simulink model "test"  (R2023a)
settings: Solver=ode1  StartTime=0.0  StopTime=inf  FixedStep=0.002  RelTol=1e-3  EnableMultiTasking=on
undefined symbols (not defined in the file or in its folder): HIL
libraries: quarc_library x18, simulink x1
settings Model: ExtModeTrigDuration=10000  Creator=bajdus  LastModifiedBy=bajdus
settings SolverCC: AlgebraicLoopSolver=TrustRegion  PositivePriorityOrder=on
settings DataIOCC: ReturnWorkspaceOutputs=off
settings DebuggingCC: UnconnectedInputMsg=warning  UnconnectedOutputMsg=warning  UnconnectedLineMsg=warning  ArithmeticOperatorsInVariantConditions=warning
settings HardwareCC: ProdBitPerLong=64  ProdLargestAtomicInteger=LongLong  ProdLargestAtomicFloat=Double  ProdLongLongMode=on  ProdHWDeviceType=ARM Compatible->ARM 64-bit (LP64)
settings ModelReferenceCC: EnableRefExpFcnMdlSchedulingChecks=on
settings SFSimCC: SimUseLocalCustomCode=off  CustomCodeUndefinedFunction=UseInterfaceOnly
settings RTWCC: Description=QUARC Linux QCar2 Target Using Toolchain  SystemTargetFile=quarc_linux_qcar2.tlc  TemplateMakefile=quarc_default_tmf  RTWUseLocalCustomCode=off  Toolchain=QUARC linux_qcar2 | gmake (64-bit Windows)  BuildConfiguration=Faster Runs
settings CodeAppCC: StateflowObjectComments=on
settings STFCustomTargetCC: SystemTargetFile=quarc_linux_qcar2.tlc
settings GRTTargetCC: ParMdlRefBuildCompliant=off  CompOptLevelCompliant=off  CombineOutputUpdateFcns=off  MatFileLogging=off  CPPClassGenCompliant=off  GRTInterface=on  ExtMode=on  ExtModeMexFile=quarc_comm  ExtModeMexArgs='-w -d /tmp -uri %u', 'tcpip://192.168.1.126:17001'
settings ConfigComp: CovMetricSettings=dswe

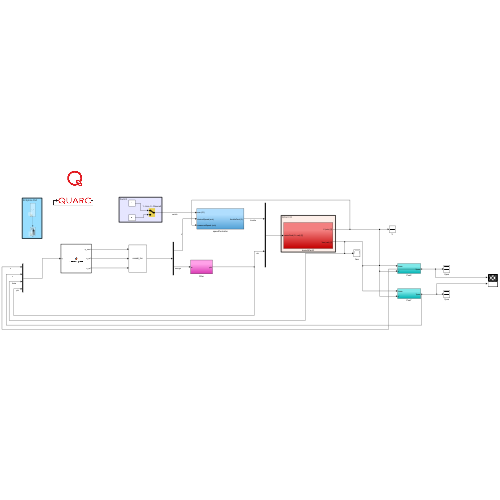
[thumbnail: Simulink's stored preview of the top-level diagram]
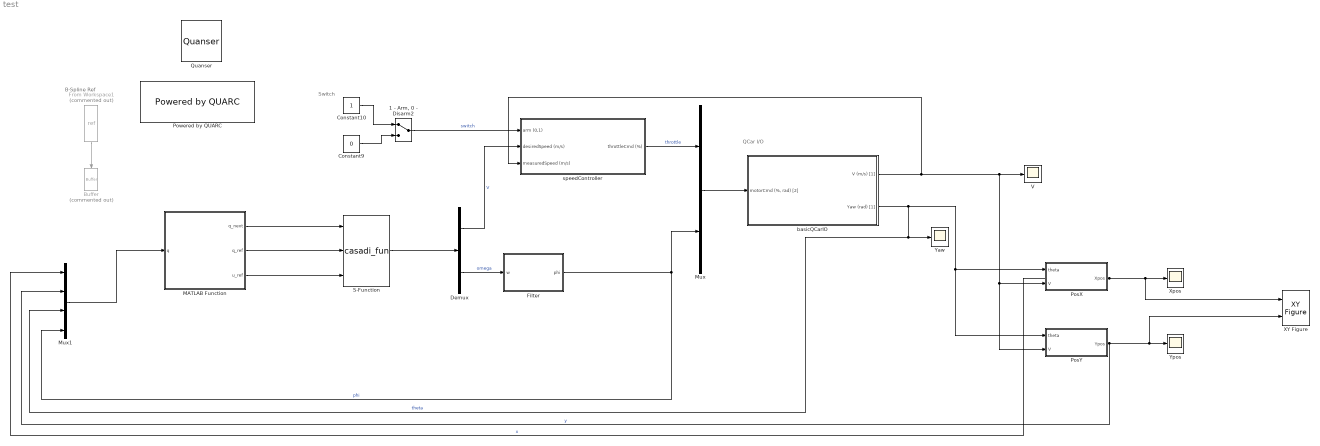
== system test ==
  note: QCar I/O
  note: Switch
  note: B-Spline Ref
  "1 - Arm, 0 - Disarm2" : ManualSwitch
  Buffer : Buffer  Commented=on  N=54  OutputFrames=off
  Constant10 : Constant
  Constant9 : Constant  Value=0
  Demux : Demux  Outputs=2
  Filter : Subsystem
  From Workspace1 : FromWorkspace  Commented=on  VariableName=ref  SampleTime=0.1  ZeroCross=off
  MATLAB Function : MATLAB Function  TreatAsAtomicUnit=on
  Mux : Mux  Inputs=2
  Mux1 : Mux
  PosX : Subsystem
  PosY : Subsystem
  Powered by QUARC : quarc_library/Logos/Powered by QUARC
  Quanser : quarc_library/Logos/Quanser
  S-Function : S-Function  FunctionName=casadi_fun  Parameters='nmpc_oncar.casadi','nmpc_oncar'  SFunctionDeploymentMode=off  EnableBusSupport=off
  V : Scope
  XY Figure : quarc_library/Sinks/Figures/XY Figure  figure_mode=Use figure window  figure_tag=figure1  axes_tag=axes1  plot_mode=Time-based  minimum_x=-5  maximum_x=5  minimum_y=-5  maximum_y=5  buffer_size=1000000  update_rate=100  initial_position="1.8          41.8         439.2         331.2"  initial_visibility=off  sample_time=-1
      settings: SourceProductName=QUARC Targets
  Xpos : Scope
  Yaw : Scope
  Ypos : Scope
  basicQCarIO : Subsystem
  speedController : Subsystem
  wires:
  Mux/1 -> basicQCarIO/1("motorCmd (%, rad) [2]")
  "1 - Arm, 0 - Disarm2"/1 -> speedController/1(arm (0,1))  "switch"
  Constant10/1 -> "1 - Arm, 0 - Disarm2"/1
  speedController/1(throttleCmd (%)) -> Mux/1  "throttle"
  basicQCarIO/1(V (m/s) [1]) -> speedController/3(measuredSpeed (m/s)), V/1, PosX/2(V), PosY/2(V)
  Constant9/1 -> "1 - Arm, 0 - Disarm2"/2
  PosX/1(Xpos) -> XY Figure/1, Xpos/1, Mux1/1  "x"
  PosY/1(Ypos) -> XY Figure/2, Ypos/1, Mux1/2  "y"
  basicQCarIO/2(Yaw (rad) [1]) -> Mux1/3, Yaw/1, PosY/1(theta), PosX/1(theta)  "theta"
  Filter/1(phi) -> Mux1/4, Mux/2  "phi"
  Demux/1 -> speedController/2(desiredSpeed (m/s))  "V"
  Demux/2 -> Filter/1(w)  "omega"
  From Workspace1/1 -> Buffer/1
  Mux1/1 -> MATLAB Function/1(q)
  S-Function/1 -> Demux/1
  MATLAB Function/1(q_next) -> S-Function/1
  MATLAB Function/2(q_ref) -> S-Function/2
  MATLAB Function/3(u_ref) -> S-Function/3

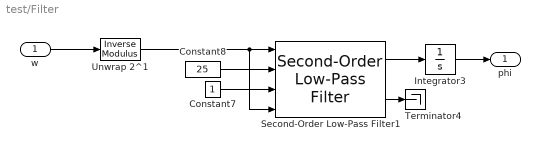
== system test/Filter ==
  w : Inport
  Constant7 : Constant
  Constant8 : Constant  Value=25
  Integrator3 : Integrator
  Second-Order Low-Pass Filter1 : quarc_library/Continuous/Second-Order Low-Pass Filter  params_source=External (input ports)  input_width=1  input_zeta=1  input_init=0
  Terminator4 : Terminator
  Unwrap 2^1 : quarc_library/Discontinuities/Inverse Modulus  modulus=16777215  output_derivative=off  output_revolutions=off  max_x=Inf  min_x=-Inf
  phi : Outport
  wires:
  Constant8/1 -> Second-Order Low-Pass Filter1/2
  Constant7/1 -> Second-Order Low-Pass Filter1/3
  Second-Order Low-Pass Filter1/1 -> Integrator3/1
  Unwrap 2^1/1 -> Second-Order Low-Pass Filter1/4, Second-Order Low-Pass Filter1/1
  w/1 -> Unwrap 2^1/1
  Second-Order Low-Pass Filter1/2 -> Terminator4/1
  Integrator3/1 -> phi/1

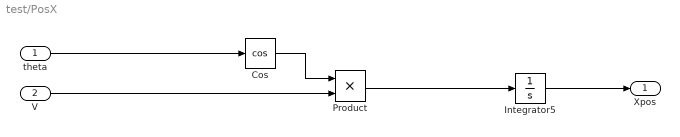
== system test/PosX ==
  theta : Inport
  V : Inport  Port=2
  Cos : Trigonometry  Operator=cos
  Integrator5 : Integrator
  Product : Product
  Xpos : Outport
  wires:
  Cos/1 -> Product/1
  theta/1 -> Cos/1
  V/1 -> Product/2
  Integrator5/1 -> Xpos/1
  Product/1 -> Integrator5/1

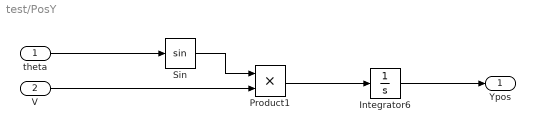
== system test/PosY ==
  theta : Inport
  V : Inport  Port=2
  Integrator6 : Integrator
  Product1 : Product
  Sin : Trigonometry
  Ypos : Outport
  wires:
  theta/1 -> Sin/1
  V/1 -> Product1/2
  Sin/1 -> Product1/1
  Integrator6/1 -> Ypos/1
  Product1/1 -> Integrator6/1

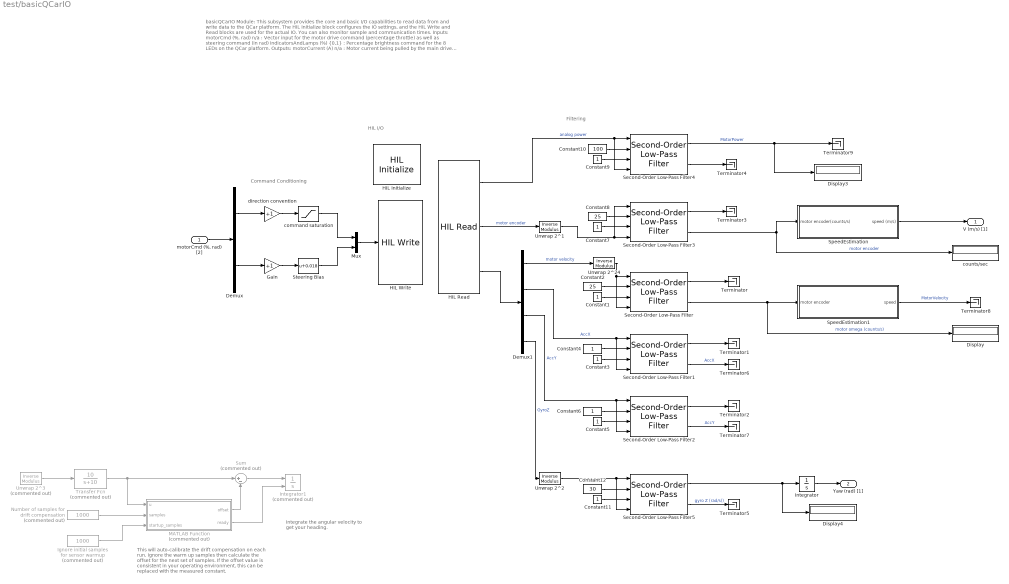
== system test/basicQCarIO ==
  note: Filtering
  note: basicQCarIO Module:
      |
      | This subsystem provides the core and basic I/O capabilities to read data from and write data to the QCar platform. The HIL Initialize block configures the IO settings, and the HIL Write and Read blocks are used for the actual IO. You can also monitor sample and communication times.
      |
      | Inputs:
      | motorCmd (%, rad) n/a : Vector input for the motor drive command (percentage throttle) as well as steering command (in rad)
      | indicatorsAndLamps (%) {0,1} : Percentage brightness command for the 8 LEDs on the QCar platform.
      |
      | Outputs:
      | motorCurrent (A) n/a : Motor current being pulled by the main drive motor
      | batteryVoltage (V) {0, 12.6} : Current battery voltage reading
      | motorSpeed (counts/s) n/a : Drive motor speed measured using an encoder (do not confuse with wheel speed as this measurement is at the drive shaft)
  note: Command Conditioning
  note: HIL I/O
  note: Integrate the angular velocity to
      | get your heading.
  note: This will auto-calibrate the drift compensation
      | on each run. Ignore the warm up samples
      | then calculate the offset for the next set of samples.
      | If the offset value is consistent in your operating
      | environment, this can be replaced with the measured
      | constant.
  "motorCmd (%, rad) [2]" : Inport
  Constant{1,3..7,9,11} (8 alike) : Constant
  Constant10 : Constant  Value=100
  Constant12 : Constant  Value=30
  Constant2 : Constant  Value=25
  Constant8 : Constant  Value=25
  Demux : Demux  Outputs=2
  Demux1 : Demux
  Display : Display
  Display3 : Display
  Display4 : Display
  Gain : Gain  Gain=+1
  HIL Initialize : quarc_library/Data Acquisition/Generic/Configuration/HIL Initialize  object_name=HIL-2  board_type=qcar2  board_number=0  board_options=gyro_fs=250;gyro_rate=500;gyro_bw=125;gyro_ord=3;accel_fs=16;accel_rate=1000;accel_bw=250;accel_ord=3;temp_bw=4000;enc0_dir=0;enc1_dir=0;enc2_dir=0;steer_bias=0.05;  exclusive=off  active=on  hardware_clocks=[]  clock_modes=[]  initial_clock_frequencies=[]  set_clock_params_at_start=off  set_clock_params_at_switch_in=off  set_clock_frequencies_at_start=off  set_clock_frequencies_at_switch_in=off  analog_input_channels=[0:4]  analog_input_configurations=[]  analog_input_maximums=[3.3]  analog_input_minimums=[0]  set_analog_input_params_at_start=off  set_analog_input_params_at_switch_in=off  analog_output_channels=[]  analog_output_maximums=[]  analog_output_minimums=[]  initial_analog_outputs=[]  final_analog_outputs=[]  watchdog_analog_outputs=[]  set_analog_output_params_at_start=off  set_analog_output_params_at_switch_in=off  set_analog_outputs_at_start=off  set_analog_outputs_at_switch_in=off  set_analog_outputs_at_terminate=off  set_analog_outputs_at_switch_out=off  set_analog_outputs_on_watchdog=off  digital_input_channels=[0:14]  digital_output_channels=[11:26]  digital_output_configuration=[]  initial_digital_outputs=[0]  final_digital_outputs=[0]  watchdog_digital_outputs=[0]  set_digital_output_params_at_start=off  set_digital_output_params_at_switch_in=off  set_digital_outputs_at_start=on  set_digital_outputs_at_switch_in=off  set_digital_outputs_at_terminate=on  set_digital_outputs_at_switch_out=off  set_digital_outputs_on_watchdog=off  encoder_channels=[0:2]  quadrature=[4]  encoder_filter_frequency=100e6/1  initial_encoder_counts=[0]  set_encoder_params_at_start=on  set_encoder_params_at_switch_in=off  set_encoder_counts_at_start=on  set_encoder_counts_at_switch_in=off  pwm_channels=[0:1]  pwm_modes=[0]  pwm_frequency=180e6/4096  pwm_configuration=[0]  pwm_alignment=[0]  pwm_polarity=[1]  pwm_leading_deadband=[]  pwm_trailing_deadband=[]  initial_pwm_outputs=[0]  final_pwm_outputs=[0]  watchdog_pwm_outputs=[0]  set_pwm_params_at_start=on  set_pwm_params_at_switch_in=off  set_pwm_outputs_at_start=on  set_pwm_outputs_at_switch_in=off  set_pwm_outputs_at_terminate=on  set_pwm_outputs_at_switch_out=off  set_pwm_outputs_on_watchdog=off  other_output_channels=[1000 11000]  initial_other_outputs=[0]  final_other_outputs=[0]  watchdog_other_outputs=[0]  set_other_outputs_at_start=on  set_other_outputs_at_switch_in=off  set_other_outputs_at_terminate=on  set_other_outputs_at_switch_out=off  set_other_outputs_on_watchdog=off
  HIL Read : quarc_library/Data Acquisition/Generic/Immediate I//O/HIL Read  object_name=HIL-2  analog_channels=[4]  encoder_channels=[0]  digital_channels=[]  other_channels=[14000 4000:4001 3002]  sample_time=qc_get_step_size  active=on  vector_output=on  data_type_mode=Inherit via back propagation  encoder_data_type=double  digital_data_type=boolean
  HIL Write : quarc_library/Data Acquisition/Generic/Immediate I//O/HIL Write  object_name=HIL-2  analog_channels=[]  pwm_channels=[]  digital_channels=[]  other_channels=[11000 1000]  sample_time=qc_get_step_size  active=off  vector_input=on
  Ignore initial samples for sensor warmup : Constant  Commented=on  Value=1000
  Integrator : Integrator
  Integrator1 : Integrator  Commented=on  ExternalReset=rising
  MATLAB Function : MATLAB Function  Commented=on  TreatAsAtomicUnit=on
  Mux : Mux  Inputs=2
  Number of samples for drift compensation : Constant  Commented=on  Value=1000
  Second-Order Low-Pass Filter{,1..5} (6 alike) : quarc_library/Continuous/Second-Order Low-Pass Filter  params_source=External (input ports)  input_width=1  input_zeta=1  input_init=0
  SpeedEstimation : Subsystem
  SpeedEstimation1 : Subsystem
  Steering Bias : Bias  Bias=0.018  SaturateOnIntegerOverflow=off
  Sum : Sum  Commented=on  Inputs=|+-
  Terminator{,1..9} (10 alike) : Terminator
  Transfer Fcn : TransferFcn  Commented=on  Numerator=[10]  Denominator=[1 10]
  Unwrap 2^1 : quarc_library/Discontinuities/Inverse Modulus  modulus=16777215  output_derivative=off  output_revolutions=off  max_x=Inf  min_x=-Inf
  Unwrap 2^2 : quarc_library/Discontinuities/Inverse Modulus  modulus=16777215  output_derivative=off  output_revolutions=off  max_x=Inf  min_x=-Inf
  Unwrap 2^24 : quarc_library/Discontinuities/Inverse Modulus  modulus=16777215  output_derivative=off  output_revolutions=off  max_x=Inf  min_x=-Inf
  Unwrap 2^3 : quarc_library/Discontinuities/Inverse Modulus  Commented=on  modulus=16777215  output_derivative=off  output_revolutions=off  max_x=Inf  min_x=-Inf
  command saturation : Saturate  UpperLimit=0.25  LowerLimit=-0.25
  counts/sec : Display
  direction convention : Gain  Gain=+1
  V (m/s) [1] : Outport  VectorParamsAs1DForOutWhenUnconnected=off
  Yaw (rad) [1] : Outport  Port=2  VectorParamsAs1DForOutWhenUnconnected=off
  wires:
  Constant2/1 -> Second-Order Low-Pass Filter/2
  Unwrap 2^24/1 -> Second-Order Low-Pass Filter/4, Second-Order Low-Pass Filter/1
  Demux/2 -> Gain/1
  direction convention/1 -> command saturation/1
  "motorCmd (%, rad) [2]"/1 -> Demux/1
  Second-Order Low-Pass Filter/1 -> Terminator/1
  Second-Order Low-Pass Filter/2 -> Display/1, SpeedEstimation1/1(motor encoder)  "motor omega (counts/s)"
  Constant1/1 -> Second-Order Low-Pass Filter/3
  Demux/1 -> direction convention/1
  Gain/1 -> Steering Bias/1
  Constant7/1 -> Second-Order Low-Pass Filter3/3
  Constant8/1 -> Second-Order Low-Pass Filter3/2
  Mux/1 -> HIL Write/1
  command saturation/1 -> Mux/1
  Steering Bias/1 -> Mux/2
  Unwrap 2^1/1 -> Second-Order Low-Pass Filter3/1, Second-Order Low-Pass Filter3/4
  SpeedEstimation/1(speed (m/s)) -> V (m/s) [1]/1
  Demux1/1 -> Unwrap 2^24/1  "motor velocity"
  SpeedEstimation1/1(speed) -> Terminator8/1  "MotorVelocity"
  Second-Order Low-Pass Filter1/1 -> Terminator1/1
  Constant3/1 -> Second-Order Low-Pass Filter1/3
  Constant4/1 -> Second-Order Low-Pass Filter1/2
  Second-Order Low-Pass Filter2/1 -> Terminator2/1
  Constant5/1 -> Second-Order Low-Pass Filter2/3
  Constant6/1 -> Second-Order Low-Pass Filter2/2
  Second-Order Low-Pass Filter2/2 -> Terminator7/1  "AccY"
  Demux1/2 -> Second-Order Low-Pass Filter1/4, Second-Order Low-Pass Filter1/1  "AccX"
  Demux1/3 -> Second-Order Low-Pass Filter2/4, Second-Order Low-Pass Filter2/1  "AccY"
  HIL Read/3 -> Demux1/1
  HIL Read/1 -> Second-Order Low-Pass Filter4/4, Second-Order Low-Pass Filter4/1  "analog power"
  Second-Order Low-Pass Filter4/2 -> Terminator4/1
  Constant9/1 -> Second-Order Low-Pass Filter4/3
  Constant10/1 -> Second-Order Low-Pass Filter4/2
  Second-Order Low-Pass Filter4/1 -> Terminator9/1, Display3/1  "MotorPower"
  Constant12/1 -> Second-Order Low-Pass Filter5/2
  Constant11/1 -> Second-Order Low-Pass Filter5/3
  Second-Order Low-Pass Filter5/2 -> Terminator5/1  "gyro Z (rad/s))"
  Second-Order Low-Pass Filter5/1 -> Display4/1, Integrator/1
  Unwrap 2^2/1 -> Second-Order Low-Pass Filter5/4, Second-Order Low-Pass Filter5/1
  Number of samples for drift compensation/1 -> MATLAB Function/2(samples)
  Ignore initial samples for sensor warmup/1 -> MATLAB Function/3(startup_samples)
  MATLAB Function/1(offset) -> Sum/2
  MATLAB Function/2(ready) -> Integrator1/2
  Sum/1 -> Integrator1/1
  Second-Order Low-Pass Filter3/1 -> Terminator3/1
  Second-Order Low-Pass Filter3/2 -> counts/sec/1, SpeedEstimation/1(motor encoder(counts/s))  "motor encoder"
  Transfer Fcn/1 -> MATLAB Function/1(u), Sum/1
  Unwrap 2^3/1 -> Transfer Fcn/1
  Demux1/4 -> Unwrap 2^2/1  "GyroZ"
  Integrator/1 -> Yaw (rad) [1]/1
  HIL Read/2 -> Unwrap 2^1/1  "motor encoder"
  Second-Order Low-Pass Filter1/2 -> Terminator6/1  "AccX"

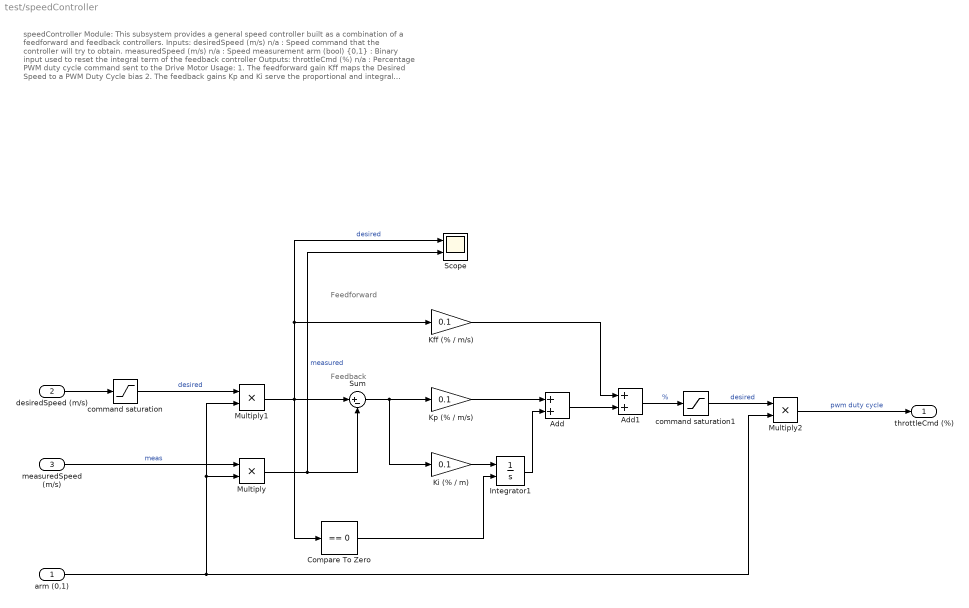
== system test/speedController ==
  note: Feedforward
  note: Feedback
  note: speedController Module:
      |
      | This subsystem provides a general speed controller built as a combination of a feedforward and feedback controllers.
      |
      | Inputs:
      | desiredSpeed (m/s) n/a : Speed command that the controller will try to obtain.
      | measuredSpeed (m/s) n/a : Speed measurement
      | arm (bool) {0,1} : Binary input used to reset the integral term of the feedback controller
      |
      | Outputs:
      | throttleCmd (%) n/a : Percentage PWM duty cycle command sent to the Drive Motor
      |
      | Usage:
      | 1. The feedforward gain Kff maps the Desired Speed to a PWM Duty Cycle bias
      | 2. The feedback gains Kp and Ki serve the proportional and integral terms to output corrections to the PWM Duty Cycle so as to regulate the desired speed.
  arm (0,1) : Inport
  desiredSpeed (m/s) : Inport  Port=2
  measuredSpeed (m/s) : Inport  Port=3
  Add : Sum
  Add1 : Sum
  Compare To Zero : simulink/Logic and Bit Operations/Compare To Zero  relop===  OutDataTypeStr=boolean
  Integrator1 : Integrator  ExternalReset=either  LimitOutput=on  UpperSaturationLimit=0.4  LowerSaturationLimit=-0.4
  Kff (% / m/s) : Gain  Gain=0.1
  "Ki (% / m) " : Gain  Gain=0.1
  Kp (% / m/s) : Gain  Gain=0.1
  Multiply : Product
  Multiply1 : Product
  Multiply2 : Product
  Scope : Scope  NumInputPorts=2
  Sum : Sum  Inputs=|+-
  command saturation : Saturate  UpperLimit=0.8  LowerLimit=-0.8
  command saturation1 : Saturate
  throttleCmd (%) : Outport  VectorParamsAs1DForOutWhenUnconnected=off
  wires:
  command saturation/1 -> Multiply1/1  "desired"
  arm (0,1)/1 -> Multiply1/2, Multiply/2, Multiply2/2
  measuredSpeed (m/s)/1 -> Multiply/1  "meas"
  Multiply/1 -> Sum/2, Scope/2  "measured"
  Add/1 -> Add1/2
  Multiply1/1 -> Compare To Zero/1, Sum/1, Kff (% / m/s)/1, Scope/1  "desired"
  Integrator1/1 -> Add/2
  Multiply2/1 -> throttleCmd (%)/1  "pwm duty cycle"
  Kp (% / m/s)/1 -> Add/1
  Compare To Zero/1 -> Integrator1/2
  Kff (% / m/s)/1 -> Add1/1
  Sum/1 -> "Ki (% / m) "/1, Kp (% / m/s)/1
  "Ki (% / m) "/1 -> Integrator1/1
  desiredSpeed (m/s)/1 -> command saturation/1
  command saturation1/1 -> Multiply2/1  "desired"
  Add1/1 -> command saturation1/1  "%"

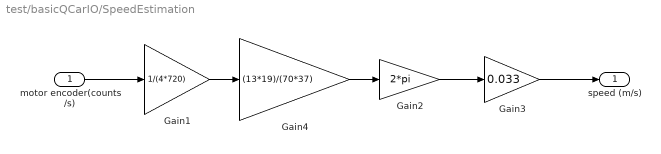
== system test/basicQCarIO/SpeedEstimation ==
  motor encoder(counts/s) : Inport
  Gain1 : Gain  Gain=1/(4*720)
  Gain2 : Gain  Gain=2*pi
  Gain3 : Gain  Gain=0.033
  Gain4 : Gain  Gain=(13*19)/(70*37)
  speed (m/s) : Outport
  wires:
  motor encoder(counts/s)/1 -> Gain1/1
  Gain1/1 -> Gain4/1
  Gain2/1 -> Gain3/1
  Gain4/1 -> Gain2/1
  Gain3/1 -> speed (m/s)/1

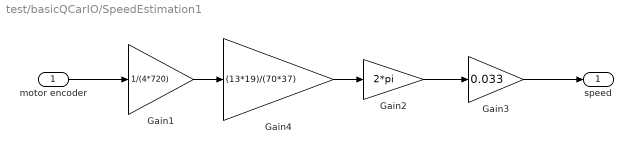
== system test/basicQCarIO/SpeedEstimation1 ==
  motor encoder : Inport
  Gain1 : Gain  Gain=1/(4*720)
  Gain2 : Gain  Gain=2*pi
  Gain3 : Gain  Gain=0.033
  Gain4 : Gain  Gain=(13*19)/(70*37)
  speed : Outport
  wires:
  motor encoder/1 -> Gain1/1
  Gain1/1 -> Gain4/1
  Gain2/1 -> Gain3/1
  Gain4/1 -> Gain2/1
  Gain3/1 -> speed/1

== matlab function test/MATLAB Function ==
  data: q input; q_next output; q_ref output; u_ref output
function [q_next, q_ref, u_ref] = discrete_plant(q)
    persistent idx q_ref_internal;

    if isempty(idx)
        idx = 1;
    end

    if isempty(q_ref_internal)
        q_ref_internal = zeros(4,1);
    end

    % Parameters
    Npred = 12;
    l = 0.256;
    L = l;
    Delta = 0.35;
    dt = 0.1; 
    
    %% Next state
    % x = q(1);
    % y = q(2);
    % theta = q(3);
    % phi = q(4);
    % 
    % v = u(1); 
    % omega = u(2);  
    % 
    % % Discretized system dynamics
    % x_next = x + dt * (v * cos(theta));  
    % y_next = y + dt * (v * sin(theta)); 
    % theta_next = theta + dt * (v / l * tan(phi));  
    % phi_next = phi + dt * omega; 

    % q_next = [x_next; y_next; theta_next; phi_next];
    q_next = zeros(4,1);
    q_next(1,1) = q(1);
    q_next(2,1) = q(2);
    q_next(3,1) = q(3);
    q_next(4,1) = q(4);
    
    %% Reference    
    % spline
    % ref = reshape(ref,[9,Npred+1]);
    % xr = ref(2, :);
    % yr = ref(3, :);
    % dddxr = ref(4, :);
    % dddyr = ref(5, :);
    % ddxr = ref(6, :);
    % ddyr = ref(7, :);
    % dxr = ref(8, :);
    % dyr = ref(9, :);

    % circle
    t = 0:dt:60;  
    alpha   = 5;
    beta    = 5;
    ang     = 0.2;
    xr = alpha*cos(ang*t);      dxr = -alpha*ang*sin(ang*t);    ddxr = -alpha*ang*ang*cos(ang*t);       dddxr = alpha*ang*ang*ang*sin(ang*t);
    yr = beta*sin(ang*t);       dyr = beta*ang*cos(ang*t);      ddyr = -beta*ang*ang*sin(ang*t);        dddyr = -beta*ang*ang*ang*cos(ang*t);

    Vr = sqrt(dxr.^2 + dyr.^2);
    omegar  = l * Vr .* ((dddyr.*dxr - dddxr.*dyr).*Vr.*Vr - 3 * (ddyr.*dxr - ddxr.*dyr) .* (dxr.*ddxr + dyr.*ddyr)) ...
              ./ (Vr.^6 + l*l*(ddyr.*dxr - ddxr.*dyr).^2);
    
    thetar = unwrap(atan2(dyr, dxr));
    phir = atan((l*(ddyr.*dxr - ddxr.*dyr)) ./ Vr.^3);
    
    % references predefined inside here
    q_ref = zeros(4, Npred + 1);
    u_ref = zeros(2, Npred);
    idx_end = min(idx + Npred, size(t,2));

    q_ref(1, :) = xr(idx:idx_end);
    q_ref(2, :) = yr(idx:idx_end);
    q_ref(3, :) = thetar(idx:idx_end);
    q_ref(4, :) = phir(idx:idx_end);

    % q_ref(1, :) = xr;
    % q_ref(2, :) = yr;
    % q_ref(3, :) = thetar;
    % q_ref(4, :) = phir;

    % q_ref_internal = [xr; yr; thetar; phir];
    % q_ref = q_ref_internal;
    
    % u_ref(1, :) = Vr(1:Npred);
    % u_ref(2, :) = omegar(1:Npred);
    u_ref(1, :) = Vr(idx:idx_end-1);
    u_ref(2, :) = omegar(idx:idx_end-1);

    idx = idx + 1;
end

== matlab function test/basicQCarIO/MATLAB Function ==
  settings: updateMethod=DISCRETE
  data: u input; offset output; samples input; ready output; startup_samples input
function [offset, ready] = fcn(u, samples, startup_samples)

persistent sample_sum;
persistent remaining_samples;
persistent last_offset;
persistent last_ready;
persistent remaining_startup_samples;

if isempty(sample_sum)
    sample_sum = 0;
    remaining_samples = samples;
    remaining_startup_samples = startup_samples;
    last_offset = 0;
    last_ready = 0;
end

if (remaining_startup_samples > 0)
    remaining_startup_samples = remaining_startup_samples - 1;
else
    if (remaining_samples > 0) && (samples > 0)
        sample_sum = sample_sum + u;
        remaining_samples = remaining_samples - 1;

        if remaining_samples == 0
            last_offset = sample_sum/samples;
            last_ready = 1;
        end
    end
end

offset = last_offset;
ready = last_ready;
